simulink model "example_simulink_RobotinoHardware"  (Simulink 7.0)
settings: Solver=FixedStepDiscrete  SolverMode=SingleTasking  StartTime=0.0  StopTime=inf  FixedStep=100  MaxStep=1  RelTol=1e-3
libraries: lib_robotinohardware x36, simulink x7
settings Model: Creator=verbeek  LastModifiedBy=verbeek
settings DebuggingCC: SaveWithParameterizedLinksMsg=none  SignalResolutionControl=TryResolveAllWithWarning  MultiTaskDSMMsg=warning  MultiTaskCondExecSysMsg=none
settings RTWCC: IncludeERTFirstTime=on
settings GRTTargetCC: TargetFcnLib=ansi_tfl_tmw.mat

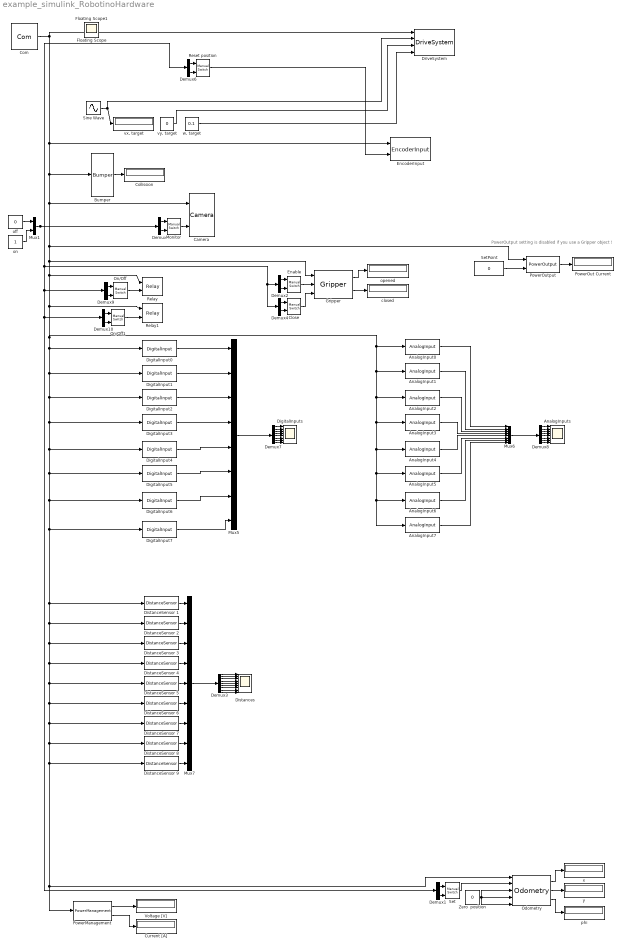
== system example_simulink_RobotinoHardware ==
  note: PowerOutput setting is disabled
      | if you use a Gripper object !
  AnalogInput{0..7} (8 alike) : lib_robotinohardware/AnalogInput  num=0
  AnalogInputs : Scope  NumInputPorts=8
      settings: YMin=0~0~0~0~0~0~0~0  YMax=2.5~2.5~2.5~2.5~2.5~2.5~2.5~2.5  SaveName=ScopeData7
  Bumper : lib_robotinohardware/Bumper
  Camera : lib_robotinohardware/Camera
  Close : simulink/Signal Routing/Manual Switch  SystemSampleTime=-1  sw=1  action=0  varsize=off
  Collission : Display
  Com : lib_robotinohardware/Com  ip='192.168.1.241'
  Current [A] : Display
  Demux{,1..2,4,6,9..10} (7 alike) : Demux  Outputs=2
  Demux3 : Demux  Outputs=9
  Demux7 : Demux  Outputs=8
  Demux8 : Demux  Outputs=8
  DigitalInput{0..7} (8 alike) : lib_robotinohardware/DigitalInput  num=0
  DigitalInputs : Scope  NumInputPorts=8
      settings: YMin=0~0~0~0~0~0~0~0  YMax=2.5~2.5~2.5~2.5~2.5~2.5~2.5~2.5  SaveName=ScopeData6
  DistanceSensor 1 : lib_robotinohardware/DistanceSensor  num=0
  DistanceSensor 2 : lib_robotinohardware/DistanceSensor  num=1
  DistanceSensor 3 : lib_robotinohardware/DistanceSensor  num=2
  DistanceSensor 4 : lib_robotinohardware/DistanceSensor  num=3
  DistanceSensor 5 : lib_robotinohardware/DistanceSensor  num=4
  DistanceSensor 6 : lib_robotinohardware/DistanceSensor  num=5
  DistanceSensor 7 : lib_robotinohardware/DistanceSensor  num=6
  DistanceSensor 8 : lib_robotinohardware/DistanceSensor  num=7
  DistanceSensor 9 : lib_robotinohardware/DistanceSensor  num=8
  Distances : Scope  NumInputPorts=9
      settings: YMin=0~0~0~0~0~0~0~0~0  YMax=2.5~2.5~2.5~2.5~2.5~2.5~2.5~2.5~2.5
  DriveSystem : lib_robotinohardware/DriveSystem
  Enable : simulink/Signal Routing/Manual Switch  SystemSampleTime=-1  sw=0  action=0  varsize=off
  EncoderInput : lib_robotinohardware/EncoderInput
  Gripper : lib_robotinohardware/Gripper
  Monitor : simulink/Signal Routing/Manual Switch  SystemSampleTime=-1  sw=0  action=0  varsize=off
  Mux1 : Mux  Inputs=2
  Mux5 : Mux  Inputs=8
  Mux6 : Mux  Inputs=8
      settings: DisplayOption=signals
  Mux7 : Mux  Inputs=9
  Odometry : lib_robotinohardware/Odometry
  On/Off : simulink/Signal Routing/Manual Switch  SystemSampleTime=-1  sw=1  action=0  varsize=off
  On/Off1 : simulink/Signal Routing/Manual Switch  SystemSampleTime=-1  sw=1  action=0  varsize=off
  PowerManagement : lib_robotinohardware/PowerManagement
  PowerOut Current : Display
  PowerOutput : lib_robotinohardware/PowerOutput
  Relay : lib_robotinohardware/Relay  num=0
  Relay1 : lib_robotinohardware/Relay  num=1
  Reset position : simulink/Signal Routing/Manual Switch  SystemSampleTime=-1  sw=1  action=0  varsize=off
  Set : simulink/Signal Routing/Manual Switch  SystemSampleTime=-1  sw=1  action=0  varsize=off
  SetPoint : Constant  Value=0  OutDataType=sfix(16)  OutScaling=2^0
  Sine Wave : Sin  Amplitude=0.5  Bias=0.5  Frequency=0.1  SampleTime=0
  Voltage [V] : Display
  Zero  position : Constant  Value=0  OutDataType=sfix(16)  OutScaling=2^0
  closed : Display
  off : Constant  Value=0  OutDataType=sfix(16)  OutScaling=2^0
  on : Constant  OutDataType=sfix(16)  OutScaling=2^0
  opened : Display
  phi : Display
  "vx, target" : Display
  "vy, target" : Constant  Value=0  OutDataType=sfix(16)  OutScaling=2^0
  "w, target" : Constant  Value=0.1  OutDataType=sfix(16)  OutScaling=2^0
  x : Display
  y : Display
  Floating Scope : Scope
      settings: Floating=on  SaveName=ScopeData4
  Floating Scope1 : Scope
      settings: Floating=on  YMin=-1  YMax=1  SaveName=ScopeData5
  wires:
  Com/1 -> DriveSystem/1, Gripper/1, Relay/1, Relay1/1, DigitalInput0/1, DigitalInput1/1, DigitalInput2/1, DigitalInput3/1, DigitalInput4/1, DigitalInput5/1, DigitalInput6/1, DigitalInput7/1, DistanceSensor 1/1, DistanceSensor 2/1, DistanceSensor 3/1, DistanceSensor 4/1, DistanceSensor 5/1, DistanceSensor 6/1, DistanceSensor 7/1, DistanceSensor 8/1, PowerManagement/1, Odometry/1, DistanceSensor 9/1, AnalogInput0/1, AnalogInput1/1, AnalogInput2/1, AnalogInput3/1, AnalogInput4/1, AnalogInput5/1, AnalogInput6/1, AnalogInput7/1, PowerOutput/1, Camera/1, Bumper/1, EncoderInput/1
  Sine Wave/1 -> "vx, target"/1, DriveSystem/2
  Monitor/1 -> Camera/2
  "vy, target"/1 -> DriveSystem/3
  "w, target"/1 -> DriveSystem/4
  Bumper/1 -> Collission/1
  off/1 -> Mux1/1
  on/1 -> Mux1/2
  Demux/1 -> Monitor/1
  Demux/2 -> Monitor/2
  Mux1/1 -> Demux/1, Demux2/1, Demux4/1, Demux9/1, Demux1/1, Demux10/1, Demux6/1
  Demux3/1 -> Distances/1
  Demux3/2 -> Distances/2
  Demux3/3 -> Distances/3
  Demux3/4 -> Distances/4
  Demux3/5 -> Distances/5
  Demux3/6 -> Distances/6
  Demux3/7 -> Distances/7
  Demux3/8 -> Distances/8
  Demux3/9 -> Distances/9
  PowerManagement/1 -> Voltage [V]/1
  PowerManagement/2 -> Current [A]/1
  Demux1/1 -> Set/1
  Demux1/2 -> Set/2
  Zero  position/1 -> Odometry/3, Odometry/5, Odometry/4
  Demux2/1 -> Enable/1
  Demux2/2 -> Enable/2
  Enable/1 -> Gripper/2
  Demux4/1 -> Close/1
  Demux4/2 -> Close/2
  Close/1 -> Gripper/3
  Demux6/1 -> Reset position/1
  Demux6/2 -> Reset position/2
  Reset position/1 -> EncoderInput/2
  PowerOutput/1 -> PowerOut Current/1
  SetPoint/1 -> PowerOutput/2
  Demux7/1 -> DigitalInputs/1
  Demux7/2 -> DigitalInputs/2
  Demux7/3 -> DigitalInputs/3
  Demux7/4 -> DigitalInputs/4
  Demux7/5 -> DigitalInputs/5
  Demux7/6 -> DigitalInputs/6
  Demux7/7 -> DigitalInputs/7
  Demux7/8 -> DigitalInputs/8
  Demux8/1 -> AnalogInputs/1
  Demux8/2 -> AnalogInputs/2
  Demux8/3 -> AnalogInputs/3
  Demux8/4 -> AnalogInputs/4
  Demux8/5 -> AnalogInputs/5
  Demux8/6 -> AnalogInputs/6
  Demux8/7 -> AnalogInputs/7
  Demux8/8 -> AnalogInputs/8
  Mux6/1 -> Demux8/1
  Gripper/1 -> opened/1
  Gripper/2 -> closed/1
  Set/1 -> Odometry/2
  Odometry/1 -> x/1
  Odometry/2 -> y/1
  Odometry/3 -> phi/1
  Demux9/1 -> On/Off/1
  Demux9/2 -> On/Off/2
  On/Off/1 -> Relay/2
  Demux10/1 -> On/Off1/1
  Demux10/2 -> On/Off1/2
  On/Off1/1 -> Relay1/2
  AnalogInput0/1 -> Mux6/1
  AnalogInput1/1 -> Mux6/2
  AnalogInput2/1 -> Mux6/3
  AnalogInput3/1 -> Mux6/4
  AnalogInput4/1 -> Mux6/5
  AnalogInput5/1 -> Mux6/6
  AnalogInput6/1 -> Mux6/7
  AnalogInput7/1 -> Mux6/8
  DistanceSensor 1/1 -> Mux7/1
  DistanceSensor 2/1 -> Mux7/2
  DistanceSensor 3/1 -> Mux7/3
  DistanceSensor 4/1 -> Mux7/4
  DistanceSensor 5/1 -> Mux7/5
  DistanceSensor 6/1 -> Mux7/6
  DistanceSensor 7/1 -> Mux7/7
  DistanceSensor 8/1 -> Mux7/8
  DistanceSensor 9/1 -> Mux7/9
  Mux7/1 -> Demux3/1
  DigitalInput0/1 -> Mux5/1
  DigitalInput1/1 -> Mux5/2
  DigitalInput2/1 -> Mux5/3
  DigitalInput3/1 -> Mux5/4
  DigitalInput4/1 -> Mux5/5
  DigitalInput5/1 -> Mux5/6
  DigitalInput6/1 -> Mux5/7
  DigitalInput7/1 -> Mux5/8
  Mux5/1 -> Demux7/1
